simulink model "IMU_VO_Android"  (R2022a)
settings: Solver=FixedStepAuto  StartTime=0.0  StopTime=10.0  RelTol=1e-3
libraries: androiduilib x6, androidsensorlib x2, androidcommunicationlib x2, androidaudiovideolib x1, simulink x1
settings Model: Creator=The MathWorks, Inc.  LastModifiedBy=mbilal
settings SolverCC: AlgebraicLoopSolver=TrustRegion
settings OptimizationCC: EnhancedBackFolding=on  PassReuseOutputArgsThreshold=0  MaxStackSize=64  OptimizeBlockOrder=speed  DifferentSizesBufferReuse=on  OptimizationCustomize=off
settings DebuggingCC: ParameterTunabilityLossMsg=error  UnconnectedInputMsg=warning  UnconnectedOutputMsg=warning  UnconnectedLineMsg=warning  SFMachineParentedDataDiag=warning  ArithmeticOperatorsInVariantConditions=warning
settings HardwareCC: ProdBitPerPointer=32  ProdBitPerSizeT=32  ProdBitPerPtrDiffT=32  ProdLargestAtomicInteger=Long  ProdLargestAtomicFloat=Double  ProdWordSize=32  ProdHWDeviceType=ARM Compatible->ARM Cortex  UseEmbeddedCoderFeatures=off  UseSimulinkCoderFeatures=off
settings SFSimCC: CustomCodeUndefinedFunction=UseInterfaceOnly
settings RTWCC: SystemTargetFile=ert.tlc  HardwareBoard=Android Device  TLCOptions="-aInlineSetEventsForThisBaseRateFcn=TLC_FALSE -aSuppressMultiTaskScheduler=TLC_FALSE  -aRateBasedStepFcn=0"  TemplateMakefile=ert_default_tmf  GenerateReport=on  RTWVerbose=off  Toolchain=Android SDK/NDK Tools  LaunchReport=on  DLArmComputeVersion=19.05
settings CodeAppCC: ForceParamTrailComments=on  OperatorAnnotations=on
settings ERTTargetCC: ERTCustomFileBanners=off  SupportContinuousTime=on  SupportNonInlinedSFcns=on  RemoveResetFunc=off  ModelStepFunctionPrototypeControlCompliant=off

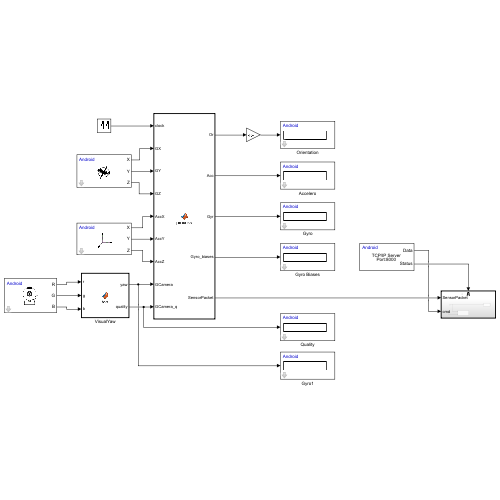
[thumbnail: Simulink's stored preview of the top-level diagram]
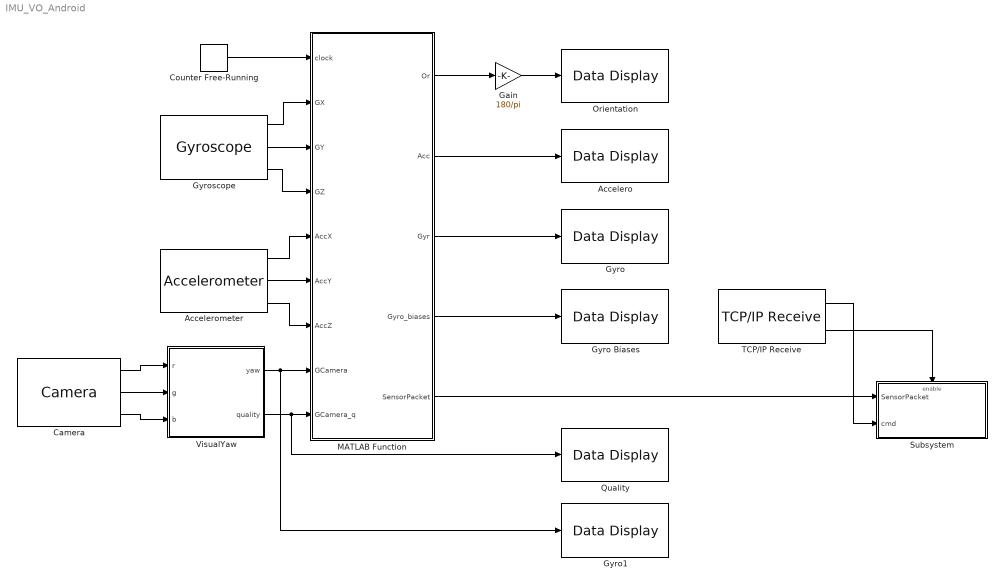
== system IMU_VO_Android ==
  Accelero : androiduilib/Data Display  DataDisplayId=IMU_VO_Android/Accelero  Format=Float  Precision=6  SimulateUsing=Code generation  blockPlatform=Android
      settings: SourceProductBaseCode=ANDROID
  Accelerometer : androidsensorlib/Accelerometer  OutputVector=off  SampleTime=0.1  BlockPlatform=Android
      settings: SourceProductBaseCode=ANDROID
  Camera : androidaudiovideolib/Camera  CameraLocation=Back  CameraResolutions=Back - 640x480  Width=640  Height=480  SampleTime=0.1  BlockPlatform=Android
      settings: SourceProductBaseCode=ANDROID
  Counter Free-Running : simulink/Sources/Counter Free-Running  NumBits=32  tsamp=0.1
  Gain : Gain  Gain=180/pi
  Gyro : androiduilib/Data Display  DataDisplayId=IMU_VO_Android/Gyro  Format=Float  Precision=6  SimulateUsing=Code generation  blockPlatform=Android
      settings: SourceProductBaseCode=ANDROID
  Gyro Biases : androiduilib/Data Display  DataDisplayId=IMU_VO_Android/Gyro_Biases  Format=Float  Precision=6  SimulateUsing=Code generation  blockPlatform=Android
      settings: SourceProductBaseCode=ANDROID
  Gyro1 : androiduilib/Data Display  DataDisplayId=IMU_VO_Android/Gyro1  Format=Float  Precision=6  SimulateUsing=Code generation  blockPlatform=Android
      settings: SourceProductBaseCode=ANDROID
  Gyroscope : androidsensorlib/Gyroscope  OutputVector=off  SampleTime=0.1  BlockPlatform=Android
      settings: SourceProductBaseCode=ANDROID
  MATLAB Function : MATLAB Function  TreatAsAtomicUnit=on
  Orientation : androiduilib/Data Display  DataDisplayId=IMU_VO_Android/Orientation  Format=Float  Precision=6  SimulateUsing=Code generation  blockPlatform=Android
      settings: SourceProductBaseCode=ANDROID
  Quality : androiduilib/Data Display  DataDisplayId=IMU_VO_Android/Quality  Format=Float  Precision=6  SimulateUsing=Code generation  blockPlatform=Android
      settings: SourceProductBaseCode=ANDROID
  Subsystem : Subsystem
  TCP/IP Receive : androidcommunicationlib/TCP//IP Receive  TCPReceiveId=IMU_VO_Android/TCP//IP_Receive  Mode_=Server  LocalServerPort_=8000  RemoteAddr_=127.0.0.1  RemoteServerPort_=25000  DataType_=uint8  DataSize_=1  SampleTime_=0.1  ClientPortBindingSelection_=off  ClientPortToBind_=35000  BlockingMode_=off  BlockTimeout_=0.1
      settings: SourceProductBaseCode=ANDROID
  VisualYaw : MATLAB Function  TreatAsAtomicUnit=on
  wires:
  Counter Free-Running/1 -> MATLAB Function/1(clock)
  Accelerometer/1 -> MATLAB Function/5(AccX)
  Accelerometer/2 -> MATLAB Function/6(AccY)
  Accelerometer/3 -> MATLAB Function/7(AccZ)
  Gyroscope/1 -> MATLAB Function/2(GX)
  Gyroscope/2 -> MATLAB Function/3(GY)
  Gyroscope/3 -> MATLAB Function/4(GZ)
  MATLAB Function/1(Or) -> Gain/1
  MATLAB Function/2(Acc) -> Accelero/1
  MATLAB Function/3(Gyr) -> Gyro/1
  MATLAB Function/4(Gyro_biases) -> Gyro Biases/1
  MATLAB Function/5(SensorPacket) -> Subsystem/1("SensorPacket ")
  TCP/IP Receive/2 -> Subsystem/Enable
  TCP/IP Receive/1 -> Subsystem/2(cmd)
  Gain/1 -> Orientation/1
  Camera/1 -> VisualYaw/1(r)
  Camera/2 -> VisualYaw/2(g)
  Camera/3 -> VisualYaw/3(b)
  VisualYaw/1(yaw) -> Gyro1/1, MATLAB Function/8(GCamera)
  VisualYaw/2(quality) -> Quality/1, MATLAB Function/9(GCamera_q)

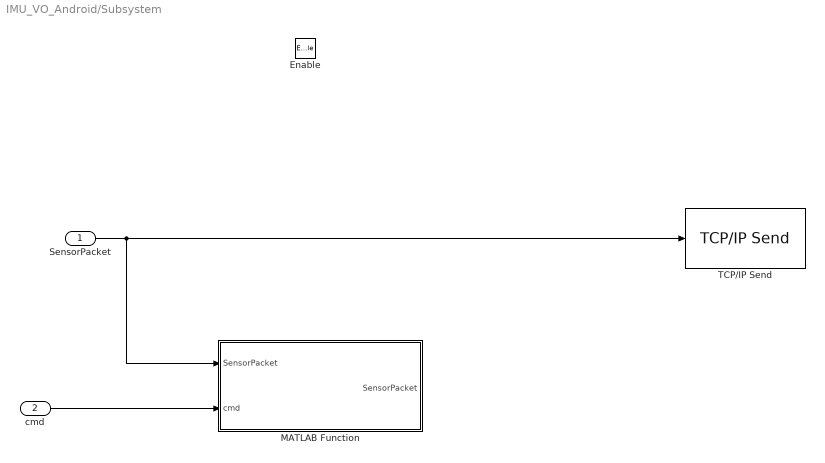
== system IMU_VO_Android/Subsystem ==
  "SensorPacket " : Inport
  cmd : Inport  Port=2
  Enable : EnablePort
  MATLAB Function : MATLAB Function  TreatAsAtomicUnit=on
  TCP/IP Send : androidcommunicationlib/TCP//IP Send  TCPSendId=IMU_VO_Android/Subsystem/TCP//IP_Send  Mode_=Server  LocalServerPort_=8000  RemoteAddr_=127.0.0.1  RemoteServerPort_=25000  ClientPortBindingSelection_=off  ClientPortToBind_=35000  BlockingMode_=off  BlockTimeout_=0.1
      settings: SourceProductBaseCode=ANDROID
  wires:
  "SensorPacket "/1 -> MATLAB Function/1("SensorPacket "), TCP/IP Send/1
  cmd/1 -> MATLAB Function/2(cmd)

== matlab function IMU_VO_Android/Subsystem/MATLAB Function ==
  data: SensorPacket input; cmd input; SensorPacket output size=[1 40]
function SensorPacket  = process(SensorPacket,cmd)
end

== matlab function IMU_VO_Android/MATLAB Function ==
  data: clock input; Or output; GX input; GY input; GZ input; AccX input; AccY input; AccZ input; Acc output; Gyr output; Gyro_biases output; SensorPacket output size=[1 40]; GCamera input; GCamera_q input
function [Or, Acc, Gyr, Gyro_biases, SensorPacket] = process(clock, GX, GY, GZ, AccX, AccY, AccZ, GCamera, GCamera_q)
% Orientation sensor is the cross product betwen Acc and Mag. Unreliable while indoors
persistent yaw;
persistent pitch;
persistent roll;
persistent biases;


if(isempty(yaw))
    yaw = double(0);
    pitch = double(0);
    roll = double(0);
    biases = [GX,GY,GZ];
end

g = sqrt(AccX^2 + AccY^2 + AccZ^2);
if(g<0.01)
    g = single(9.8);
end
Acc_pitch = double(asin(AccX/g));
Acc_roll = double(atan2(AccY,AccZ));

if(clock<50)
    biases = biases*0.99 + [GX,GY,GZ]*0.01;
end
Gyro_biases = biases;
GX = GX-biases(1);
GY = GY-biases(2);
GZ = GZ-biases(3);

GZ_q = 1-min(0.1,abs(GZ))*10;
alpha = GCamera*GZ_q;
GZ = GCamera_q*alpha + (1-alpha)*GZ;

%Rotate Gyro sensor frame to world frame
GX_w = GX + GY*sin(roll)*tan(pitch) + GZ*cos(roll)*tan(pitch);
GY_w = GY*cos(roll) - GZ*sin(roll);
GZ_w = GY*sin(roll)/cos(pitch) + GZ*cos(roll)/cos(pitch);

dt = double(0.1);
alpha = double(0.05);

if(~isnan(GX_w))
    roll = roll + double(GX_w)*dt;
    roll = roll*(1-alpha) + Acc_roll*alpha;
    roll = wrapToPi(roll);
end

if(~isnan(GY_w))
    pitch = pitch + double(GY_w)*dt;
    pitch = pitch*(1-alpha) + Acc_pitch*alpha;
    pitch = wrapToPi(pitch);
end

if(~isnan(GZ_w))
    GZwt = double(GZ_w)*dt;
    yaw = yaw + GZwt;
    yaw = wrapToPi(yaw);
end

Or = [yaw,pitch,roll];
Acc = [AccX, AccY, AccZ];
Gyr = [GX, GY, GZ];

SensorPacket = [typecast(single(yaw),'uint8'),typecast(single(pitch),'uint8'),typecast(single(roll),'uint8'),typecast(single(AccX),'uint8'),typecast(single(AccY),'uint8'),typecast(single(AccZ),'uint8'),typecast(single(GX),'uint8'),typecast(single(GY),'uint8'),typecast(single(GZ),'uint8'),typecast(single(clock),'uint8')];

end

== matlab function IMU_VO_Android/VisualYaw ==
  data: r input; g input; b input; yaw output; quality output
function [yaw,quality]  = fcn(r,g,b)
persistent img_prev;
persistent prevPoints;
persistent prevFeatures;
% persistent angle;
numPoints = 300;
    
if(isempty(img_prev))
    img_prev = cat(3,r,g,b);
    img_prev_I = im2gray(img_prev);
    prevPoints = detectSURFFeatures(img_prev_I, 'MetricThreshold', 500);
    prevPoints = selectUniform(prevPoints, numPoints, size(img_prev_I));
    prevFeatures = extractFeatures(img_prev_I, prevPoints);
%     angle = 0;
end

    Irgb = cat(3,r,g,b);
    I = im2gray(Irgb);
    currPoints   = detectSURFFeatures(I, 'MetricThreshold', 500);
    currPoints   = selectUniform(currPoints, numPoints, size(I));
    currFeatures = extractFeatures(I, currPoints);
    indexPairs = matchFeatures(prevFeatures, currFeatures, 'Unique', true);
    currPointsI = currPoints.Location(indexPairs(:,2),:);
    prevPointsI = prevPoints.Location(indexPairs(:,1),:);
    tform = estimateGeometricTransform2D(currPointsI,prevPointsI,'similarity');
    invTform = invert(tform);
    Ainv = invTform.T;

    ss = Ainv(1,2);
    sc = Ainv(1,1);
    scaleRecovered = hypot(ss,sc);
    thetaRecovered = atan2d(-ss,sc);
%     angle = angle + double(thetaRecovered);

%     img_prev_I = I;
    prevFeatures = currFeatures;
    prevPoints   = currPoints;
%     angle_o = single(angle);
    yaw = thetaRecovered*0.1745329251994329576923690768489;
    quality = min(1,length(currPointsI)/200);
